simulink model "Given_Model_Task_2"  (R2021a)
settings: Solver=VariableStepAuto  StartTime=0.0  StopTime=10.0  RelTol=1e-3
values from neighbouring files (symbols this model uses):
  A = [0 0 1 0 ... (first row only)    [Task_1.m]
  B = [0; 0; 1/mc; 1/(L*mc)]    [Task_1.m]
settings Model: Creator=jai_bhawani  LastModifiedBy=jai_bhawani

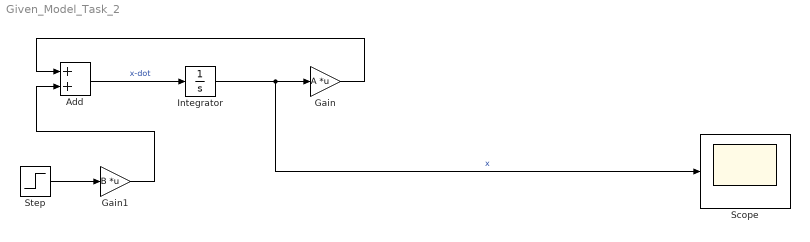
== system Given_Model_Task_2 ==
  Add : Sum
  Gain : Gain  Gain=A  Multiplication=Matrix(K*u)
  Gain1 : Gain  Gain=B  Multiplication=Matrix(K*u)
  Integrator : Integrator  InitialCondition=[0 (10*pi)/180 0 0]
  Scope : Scope
  Step : Step  Time=0  SampleTime=0
  wires:
  Add/1 -> Integrator/1  "x-dot"
  Gain1/1 -> Add/2
  Step/1 -> Gain1/1
  Gain/1 -> Add/1
  Integrator/1 -> Scope/1, Gain/1  "x"
